simulink model "bb"  (R2024a)
settings: Solver=VariableStepAuto  StartTime=0.0  StopTime=10.0  RelTol=1e-3
values from neighbouring files (symbols this model uses):
  d = 0.03    [Ball and Beam.m]    (also in bb2.m; bb3.m)
  g = -9.8    [Ball and Beam.m]    (also in bb2.m; bb3.m)
  J = 9.99e-6    (= 9.99e-06)    [Ball and Beam.m]    (also in bb2.m; bb3.m)
  L = 1.0    (= 1)    [Ball and Beam.m]    (also in bb2.m; bb3.m)
  m = 0.11    [Ball and Beam.m]    (also in bb2.m = 0.111; bb3.m)
  R = 0.015    [Ball and Beam.m]    (also in bb2.m; bb3.m)
settings Model: Creator=shukl  LastModifiedBy=shukl

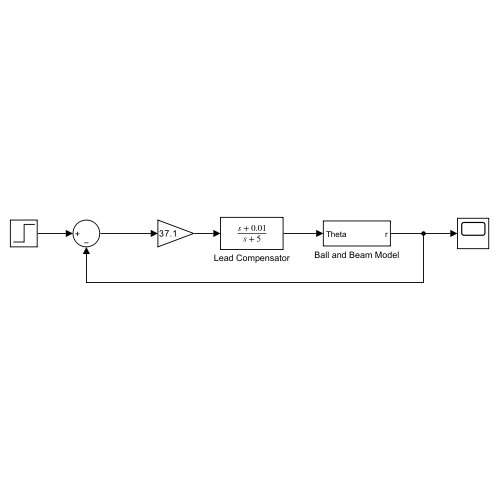
[thumbnail: Simulink's stored preview of the top-level diagram]
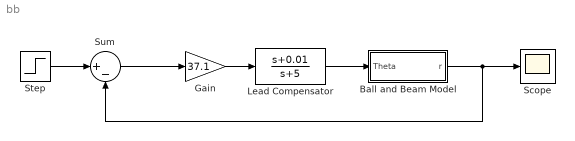
== system bb ==
  Ball and Beam Model : Subsystem
  Gain : Gain  Gain=37.1
  Lead Compensator : TransferFcn  Numerator=[1 0.01]  Denominator=[1 5]
  Scope : Scope
  Step : Step  SampleTime=0
  Sum : Sum  Inputs=|+-
  wires:
  Ball and Beam Model/1(r) -> Sum/2, Scope/1
  Lead Compensator/1 -> Ball and Beam Model/1(Theta)
  Step/1 -> Sum/1
  Sum/1 -> Gain/1
  Gain/1 -> Lead Compensator/1

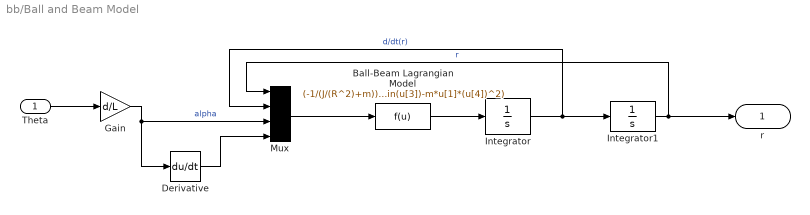
== system bb/Ball and Beam Model ==
  Theta : Inport
  Ball-Beam Lagrangian Model : Fcn  Expr=(-1/(J/(R^2)+m))*(m*g*sin(u[3])-m*u[1]*(u[4])^2)
  Derivative : Derivative
  Gain : Gain  Gain=d/L
  Integrator : Integrator
  Integrator1 : Integrator
  Mux : Mux
  r : Outport
  wires:
  Ball-Beam Lagrangian Model/1 -> Integrator/1
  Theta/1 -> Gain/1
  Integrator1/1 -> Mux/1, r/1  "r"
  Integrator/1 -> Mux/2, Integrator1/1  "d/dt(r)"
  Derivative/1 -> Mux/4
  Gain/1 -> Derivative/1, Mux/3  "alpha"
  Mux/1 -> Ball-Beam Lagrangian Model/1
